simulink model "super"  (R2018b)
settings: Solver=FixedStepAuto  StartTime=0.0  StopTime=10.0  RelTol=1e-3
libraries: sldvlib x1
settings Model: Creator=Leon Wehmeier  LastModifiedBy=Leon Wehmeier

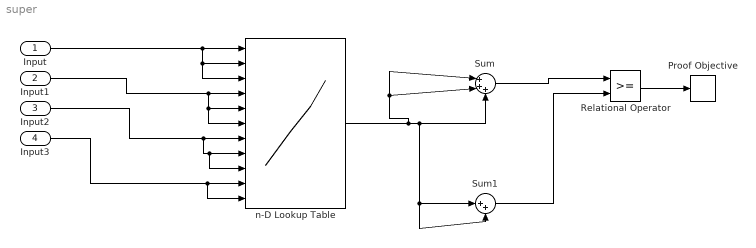
== system super ==
  Input : Inport  OutMin=0.0  OutMax=1.0  OutDataTypeStr=double
  Input1 : Inport  Port=2  OutMin=0.0  OutMax=1.0  OutDataTypeStr=double
  Input2 : Inport  Port=3  OutMin=0.0  OutMax=1.0  OutDataTypeStr=double
  Input3 : Inport  Port=4  OutMin=0.0  OutMax=1.0  OutDataTypeStr=double
  Proof Objective : sldvlib/Objectives and Constraints/Proof Objective  enabled=on  customAVTBlockType=Proof Objective  intervals=true  dispValues=on  outEnabled=off  enableStopSim=off
      settings: AttributesFormatString=%<intervals>  SourceProductName=Simulink Design Verifier  SourceProductBaseCode=DV
  Relational Operator : RelationalOperator  OutDataTypeStr=boolean  RndMeth=Simplest
  Sum : Sum  Inputs=|+++
  Sum1 : Sum  Inputs=|++
  n-D Lookup Table : Lookup_n-D  NumberOfTableDimensions=11  BreakpointsForDimension3=[5, 7]  Table=reshape(repmat([4 5 6;16 19 20;10 18 23],1,2),[3,3,2])  InternalRulePriority=Speed  OutMin=0  OutMax=1  OutDataTypeStr=double  RndMeth=Simplest  InputSameDT=on
  wires:
  Relational Operator/1 -> Proof Objective/1
  n-D Lookup Table/1 -> Sum1/1, Sum1/2, Sum/3, Sum/1, Sum/2
  Sum/1 -> Relational Operator/1
  Sum1/1 -> Relational Operator/2
  Input/1 -> n-D Lookup Table/1, n-D Lookup Table/2, n-D Lookup Table/3
  Input1/1 -> n-D Lookup Table/4, n-D Lookup Table/6, n-D Lookup Table/5
  Input2/1 -> n-D Lookup Table/7, n-D Lookup Table/9, n-D Lookup Table/8
  Input3/1 -> n-D Lookup Table/11, n-D Lookup Table/10
